simulink model "passivemodel"  (R2025b)
settings: Solver=VariableStepAuto  StartTime=0.0  StopTime=10.0  RelTol=1e-3
libraries: simulink x1
settings Model: Creator=claygrant  LastModifiedBy=wangxuanyi

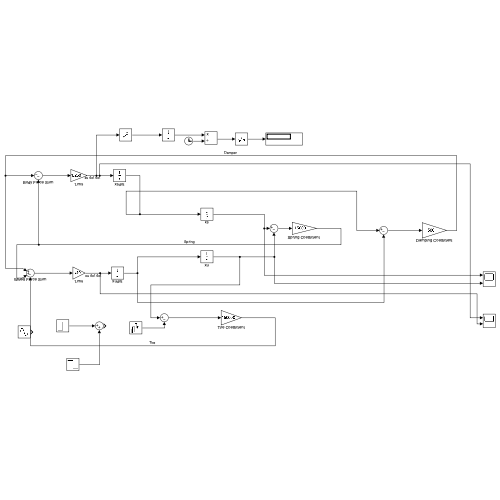
[thumbnail: Simulink's stored preview of the top-level diagram]
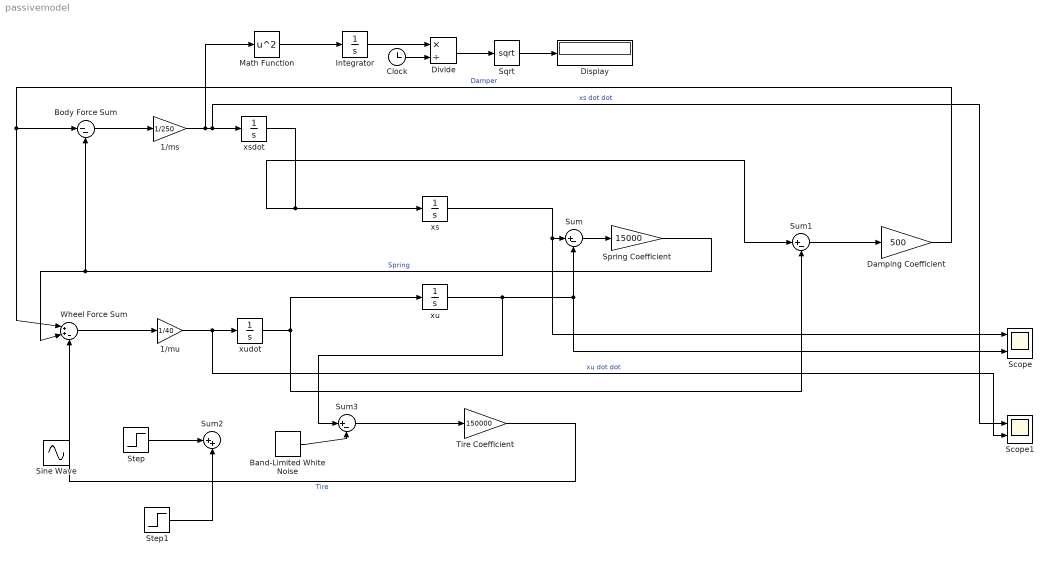
== system passivemodel ==
  1/ms : Gain  Gain=1/250
  1/mu : Gain  Gain=1/40
  Band-Limited White Noise : simulink/Sources/Band-Limited White Noise  Cov=[1e-4]  Ts=0.1  seed=[23341]
  Body Force Sum : Sum  Inputs=|--
  Clock : Clock
  Damping Coefficient : Gain  Gain=500
  Display : Display
  Divide : Product  Inputs=*/
  Integrator : Integrator
  Math Function : Math  Operator=square
  Scope : Scope  NumInputPorts=2
      settings: ActiveDisplayYMinimum=-0.14495324196355114  ActiveDisplayYMaximum=0.18422000966299806
  Scope1 : Scope  NumInputPorts=2
      settings: ActiveDisplayYMinimum=-405.36097133201582  ActiveDisplayYMaximum=494.218153062275
  Sine Wave : Sin  Amplitude=0.02  Frequency=10  SampleTime=0
  "Spring Coefficient " : Gain  Gain=15000
  Sqrt : Sqrt
  Step : Step  After=0.05  SampleTime=0
  Step1 : Step  Time=1.5  After=-0.05  SampleTime=0
  Sum : Sum  Inputs=|+-
  Sum1 : Sum  Inputs=|+-
  Sum2 : Sum  Inputs=|++
  Sum3 : Sum  Inputs=|+-
  Tire Coefficient : Gain  Gain=150000
  Wheel Force Sum : Sum  Inputs=|++-
  xs : Integrator
  xsdot : Integrator
  xu : Integrator
  xudot : Integrator
  wires:
  xs/1 -> Scope/1, Sum/1
  xu/1 -> Sum3/1, Scope/2, Sum/2
  Sum/1 -> "Spring Coefficient "/1
  xsdot/1 -> Sum1/1, xs/1
  xudot/1 -> xu/1, Sum1/2
  Sum1/1 -> Damping Coefficient/1
  Wheel Force Sum/1 -> 1/mu/1
  Body Force Sum/1 -> 1/ms/1
  1/ms/1 -> Math Function/1, Scope1/1, xsdot/1  "xs dot dot"
  1/mu/1 -> Scope1/2, xudot/1  "xu dot dot"
  "Spring Coefficient "/1 -> Wheel Force Sum/2, Body Force Sum/2  "Spring"
  Damping Coefficient/1 -> Body Force Sum/1, Wheel Force Sum/1  "Damper"
  Sum3/1 -> Tire Coefficient/1
  Tire Coefficient/1 -> Wheel Force Sum/3  "Tire"
  Step/1 -> Sum2/1
  Step1/1 -> Sum2/2
  Band-Limited White Noise/1 -> Sum3/2
  Integrator/1 -> Divide/1
  Sqrt/1 -> Display/1
  Clock/1 -> Divide/2
  Divide/1 -> Sqrt/1
  Math Function/1 -> Integrator/1
